simulink model "omega2thrust_cross"  (Simulink 9.2)
settings: Solver=FixedStepAuto  StartTime=0.0  StopTime=10.0  FixedStep=continuous_h  RelTol=1e-3  EnableMultiTasking=on
undefined symbols (not defined in the file): b, k, l
settings Model: Creator=mgreiff  LastModifiedBy=sebbe
settings DataIOCC: LimitDataPoints=off  SaveFormat=Dataset  SignalLoggingSaveFormat=Dataset
settings DebuggingCC: UnderspecifiedInitializationDetection=Simplified  MergeDetectMultiDrivingBlocksExec=error  FcnCallInpInsideContextMsg=error  StateNameClashWarn=none  SFExecutionAtInitializationDiag=warning
settings HardwareCC: ProdBitPerPointer=64  ProdBitPerSizeT=64  ProdBitPerPtrDiffT=64  ProdLargestAtomicFloat=Float  ProdIntDivRoundTo=Zero  ProdEndianess=LittleEndian  ProdWordSize=64  ProdHWDeviceType=Intel->x86-64 (Windows64)
settings ModelReferenceCC: PropagateSignalLabelsOutOfModel=on
settings GRTTargetCC: CombineOutputUpdateFcns=on  GRTInterface=off

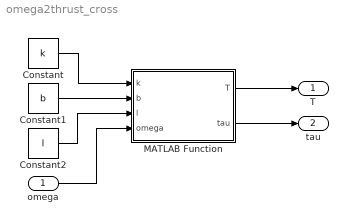
== system omega2thrust_cross ==
  omega : Inport  PortDimensions=4
  Constant : Constant  Value=k
  Constant1 : Constant  Value=b
  Constant2 : Constant  Value=l
  MATLAB Function : MATLAB Function  TreatAsAtomicUnit=on
  T : Outport  PortDimensions=1
  tau : Outport  Port=2  PortDimensions=3
  wires:
  Constant/1 -> MATLAB Function/1(k)
  omega/1 -> MATLAB Function/4(omega)
  MATLAB Function/1(T) -> T/1
  Constant2/1 -> MATLAB Function/3(l)
  Constant1/1 -> MATLAB Function/2(b)
  MATLAB Function/2(tau) -> tau/1

== matlab function MATLAB Function ==
  data: k input double; b input double; l input double; T output double; omega input double; tau output double
function [T, tau]= fcn(k, b,l, omega)
%#codegen
lc = l*0.70710678118; % Cross configuration length (1/sqrt(2))
C_t = k*lc; % Combined length and rotor constant for cross configuration
omegasq = omega.^2;

Mw = [k, k, k, k;
    -C_t, -C_t, C_t, C_t;
    -C_t, C_t, C_t, -C_t;
    -b, b, -b, b];

%Mw = [k   , k   , k  , k  ;
%      0   , -k*l, 0  , k*l;
%      -k*l, 0   , k*l, 0  ;
%      -b  , b   , -b , b  ];
Tbar = Mw*omegasq;
T = Tbar(1);
tau = Tbar(2:4);
